simulink model "main_state"  (R2021b)
settings: Solver=VariableStepAuto  StartTime=0.0  StopTime=inf  RelTol=1e-3
settings Model: Creator=User  LastModifiedBy=User

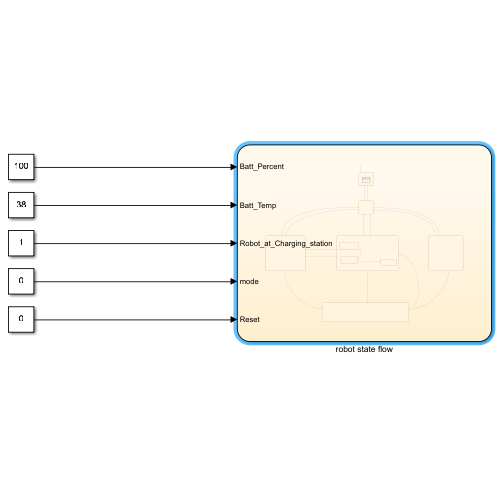
[thumbnail: Simulink's stored preview of the top-level diagram]
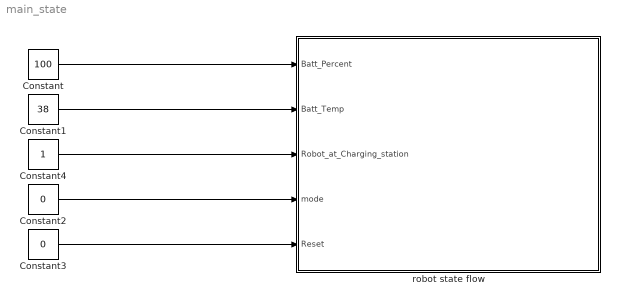
== system main_state ==
  Constant : Constant  Value=100
  Constant1 : Constant  Value=38
  Constant2 : Constant  Value=0
  Constant3 : Constant  Value=0
  Constant4 : Constant
  robot state flow : Stateflow chart  TreatAsAtomicUnit=on
  wires:
  Constant/1 -> robot state flow/1(Batt_Percent)
  Constant1/1 -> robot state flow/2(Batt_Temp)
  Constant2/1 -> robot state flow/4(mode)
  Constant3/1 -> robot state flow/5(Reset)
  Constant4/1 -> robot state flow/3(Robot_at_Charging_station)

== stateflow chart main_state/robot state flow ==
  state Reset1
    state calibrating
      state init
      state do_something
      (default) -> init
      do_something -> init : {calibrate_finish = 1}
      init -> do_something : [calibrate_finish ~= 1]
  state Stand_by
    Min_Batt = 20
    move2_C_station = 0
    Batt_Charging_Stat = 0
  state move2goal
    entry:
    done = 0;
  state charging
    Max_Batt_Temp = 40
    state check_position_robot_station
      settings: description=Check the position of the robot at the charging station.
    state Start_Batt_Charging
      if Batt_Temp > Max_Batt_Temp
      Batt_Charge_Over_Temp = 1
      end
      settings: description=Check the position of the robot at the charging station.
    state Stop_Batt_Charging
      Batt_Low_Stat = 0
      settings: description=Check the position of the robot at the charging station.
    (default) -> check_position_robot_station : {Batt_Charge_Over_Temp = 0;Emer_Charging = 0}
    check_position_robot_station -> Start_Batt_Charging : [((Robot_at_Charging_station==1&&Batt_Charge_Over_Temp==0)&&Batt_Low_Stat == 1)]{
        | Batt_Charging_Stat = 1}
    Start_Batt_Charging -> Stop_Batt_Charging : [Batt_Percent ==100]{Batt_Charging_Stat = 0}
  state Grip
    entry:
    done = 0;
  state Emergency_stop
  (default) -> Reset1 : {calibrate_finish = 0;Resume = 0;error = 0;}
  Stand_by -> Reset1 [order 1] : [Reset == 1]
  Reset1 -> Stand_by : [calibrate_finish == 1]
  move2goal -> Stand_by [order 2] : [done == 1]
  Stand_by -> Grip [order 3] : [mode == 2]
  Stand_by -> move2goal [order 2] : [mode == 1]
  Grip -> Stand_by [order 2] : [done == 1]
  charging -> Stand_by [order 1] : [Batt_Charging_Stat == 0&&Batt_Low_Stat == 0]{Batt_Low_Stat = 0}
  Stand_by -> charging [order 4] : [Batt_Percent <= Min_Batt]{Batt_Low_Stat = 1}
  charging -> move2goal [order 2] : [[Robot_at_Charging_station ~= 1]]{move2_C_station = 1}
  Emergency_stop -> charging : [[Batt_Temp < Max_Batt_Temp]]{error = 0}
  move2goal -> charging [order 3] : [Robot_at_Charging_station == 1]
  Grip -> Emergency_stop [order 1] : [error ==1]
  move2goal -> Emergency_stop [order 1] : [error ==1]
  charging -> Emergency_stop [order 3] : [Batt_Charge_Over_Temp == 1]{Batt_Charging_Stat = 0;error = 1}
  data: Batt_Percent input; calibrate_finish local; Batt_Temp input; Robot_at_Charging_station input; done local; Resume local; mode input; error local; Reset input; move2_C_station local; Emer_Charging local; Batt_Charging_Stat local; Batt_Low_Stat local; Max_Batt_Temp local; Batt_Charge_Over_Temp local; Min_Batt local
